simulink model "RudderActuatorChannel_control_linear"  (R2015a)
settings: Solver=ode4  StartTime=0.0  StopTime=2  FixedStep=sampleTime  MaxStep=1e-3  MinStep=1e-4
values from neighbouring files (symbols this model uses):
  StateControl =     [StateControl.mat]
  StateControlLinear =     [StateControlLinear.mat]
undefined symbols (not defined in the file or in its folder): C, ControlTopology, EHSV_Step, Imax, Input, Kd, Ki, Kp, L0, Load_cmd, Max_Cmd, Max_Load_TED, Max_Load_TEU, Min_Cmd, ON_OFF_hyst, OpenLoop, R, Rate_Limit, sampleTime, sigbuilder_block, StiffnessTest_Enable, StiffTest, T_ES, Theta0, Tol_SA1
undefined symbols (not defined in the file): dpLVDT, Kd_N, ramLVDT, xvLVDT
libraries: simulink x3
settings Model: SimulationMode=accelerator  Creator=Charles  LastModifiedBy=Pedro H
settings SolverCC: InitialStep=1e-4
settings DataIOCC: LimitDataPoints=off  SaveFormat=StructureWithTime  DSMLogging=off  SaveTime=off
settings OptimizationCC: ExpressionDepthLimit=2147483647  InitFltsAndDblsToZero=on
settings DebuggingCC: SaveWithParameterizedLinksMsg=none  UnderspecifiedInitializationDetection=Classic  MergeDetectMultiDrivingBlocksExec=none  SolverPrmCheckMsg=warning  InheritedTsInSrcMsg=none  FcnCallInpInsideContextMsg=UseLocalSettings  StateNameClashWarn=warning
settings ModelReferenceCC: UpdateModelReferenceTargets=IfOutOfDate
settings GRTTargetCC: TargetFcnLib=ansi_tfl_tmw.mat  CombineOutputUpdateFcns=off  GRTInterface=on

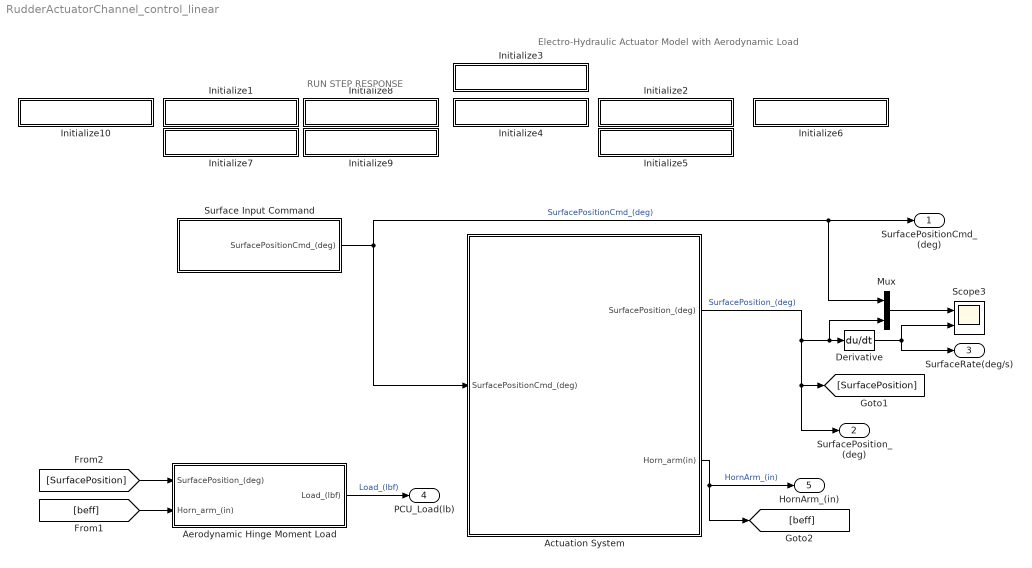
== system RudderActuatorChannel_control_linear ==
  note: RUN STEP RESPONSE
  note: Electro-Hydraulic Actuator Model with Aerodynamic Load
  Actuation System : Subsystem
  Aerodynamic Hinge Moment Load : Subsystem
  Derivative : Derivative  CoefficientInTFapproximation=1e6
  Initialize1 : Subsystem
      settings: OpenFcn=|
      | run('StepInput_CLLoad.m'),
      | set_param(bdroot,'SimulationCommand','start')
      mask Display: disp('Closed Loop - Loaded')
  Initialize10 : Subsystem
      settings: OpenFcn=|
      | run('SineInput_CLLoad.m'),
      | set_param(bdroot,'SimulationCommand','start')
      mask Display: disp('Run Sine Input')
  Initialize2 : Subsystem
      settings: OpenFcn=|
      | FreqResp_type = 0;
      | run('FrequencyResponseTest.m'),
      | set_param(bdroot,'SimulationCommand','start')
      mask Display: disp('Frequency Response')
  Initialize3 : Subsystem
      settings: OpenFcn=run('Load_Parameters.m'),
      mask Display: disp('Model Initialization')
  Initialize4 : Subsystem
      settings: OpenFcn=run('plotMaster.m')
      mask Display: disp('Plot Results')
  Initialize5 : Subsystem
      settings: OpenFcn=|
      | FreqResp_type = 1;
      | run('FrequencyResponseTest.m'),
      | set_param(bdroot,'SimulationCommand','start')
      mask Display: disp('Run EHSV Frequency Response Test')
  Initialize6 : Subsystem
      settings: OpenFcn=run('DynamicStiffnessTest.m')
      mask Display: disp('Dynamic Stiffness Test')
  Initialize7 : Subsystem
      settings: OpenFcn=|
      | run('StepInput_CLNoLoad.m'),
      | set_param(bdroot,'SimulationCommand','start')
      mask Display: disp('Closed Loop - Unloaded')
  Initialize8 : Subsystem
      settings: OpenFcn=|
      | run('StepInput_OLEHSVLoad.m'),
      | set_param(bdroot,'SimulationCommand','start')
      mask Display: disp('Open Loop - Loaded')
  Initialize9 : Subsystem
      settings: OpenFcn=|
      | run('StepInput_OLEHSVNoLoad.m'),
      | set_param(bdroot,'SimulationCommand','start')
      mask Display: disp('Open Loop - Unloaded')
  Mux : Mux  Inputs=2
  Scope3 : Scope  NumInputPorts=2
      settings: TimeRange=3.4  YMin=28.7~-5  YMax=30.8~5  SaveName=Theta
  Surface Input Command : Subsystem
  SurfacePositionCmd_(deg) : Outport
  SurfacePosition_(deg) : Outport  Port=2
  SurfaceRate(deg/s) : Outport  Port=3
  PCU_Load(lb) : Outport  Port=4
  HornArm_(in) : Outport  Port=5
  wires:
  Actuation System/1(SurfacePosition_(deg)) -> SurfacePosition_(deg)/1, [SurfacePosition], Mux/2, Derivative/1  "SurfacePosition_(deg)"
  [SurfacePosition] -> Aerodynamic Hinge Moment Load/1(SurfacePosition_(deg))
  Surface Input Command/1(SurfacePositionCmd_(deg)) -> Mux/1, SurfacePositionCmd_(deg)/1, Actuation System/1(SurfacePositionCmd_(deg))  "SurfacePositionCmd_(deg)"
  Actuation System/2(Horn_arm(in)) -> [beff], HornArm_(in)/1  "HornArm_(in)"
  [beff] -> Aerodynamic Hinge Moment Load/2(Horn_arm_(in))
  Aerodynamic Hinge Moment Load/1(Load_(lbf)) -> PCU_Load(lb)/1  "Load_(lbf)"
  Derivative/1 -> Scope3/2, SurfaceRate(deg/s)/1
  Mux/1 -> Scope3/1

== system RudderActuatorChannel_control_linear/Actuation System ==
  SurfacePositionCmd_(deg) : Inport
  Actuator : Subsystem
  Electronics System : Subsystem
  Surface Kinematics : Subsystem
  SurfacePosition_(deg) : Outport
  Horn_arm(in) : Outport  Port=2
  wires:
  [Sensors_FB] -> Electronics System/2(Sensors_FB)
  SurfacePositionCmd_(deg)/1 -> [Theta_Cmd]
  [Theta_Cmd] -> Electronics System/1(Theta_Cmd_(deg))
  Actuator/1(Xp_real_(in)) -> Surface Kinematics/1(Xp_(in))  "Xp"
  Surface Kinematics/1(ThetaPos_(deg)) -> SurfacePosition_(deg)/1
  Actuator/2(Sensors) -> [Sensors_FB]
  Surface Kinematics/2(Effective_arm_(in)) -> Horn_arm(in)/1
  Electronics System/1(Current_Cmd_(mA)) -> Actuator/1(Current_Cmd)

== system RudderActuatorChannel_control_linear/Aerodynamic Hinge Moment Load ==
  note: Aerodynamic Hinge Moment Load
  SurfacePosition_(deg) : Inport
  Horn_arm_(in) : Inport  Port=2
  1-D Lookup Table : Lookup_n-D  NumberOfTableDimensions=1  BreakpointsForDimension1=[-1 0 1]  Table=[-Max_Load_TED 0 Max_Load_TEU]  RndMeth=Simplest  InputSameDT=on
  Constant : Constant  Value=StiffnessTest_Enable
  Constant1 : Constant  Value=Load_cmd
  Divide : Product  Inputs=*/
  Gain : Gain  Gain=1/Max_Cmd
  Load Type Selector : MultiPortSwitch
  Stiffness Test Load : Sin  Amplitude=StiffTest.Sine_Amplitude  Bias=StiffTest.Sine_Bias  Frequency=StiffTest.Sine_Frequency  SampleTime=0
  Load_(lbf) : Outport
  wires:
  SurfacePosition_(deg)/1 -> Gain/1
  Constant/1 -> Load Type Selector/1
  Gain/1 -> 1-D Lookup Table/1
  Load Type Selector/1 -> Load_(lbf)/1
  Stiffness Test Load/1 -> Load Type Selector/2
  Constant1/1 -> Load Type Selector/4
  1-D Lookup Table/1 -> Divide/1
  Divide/1 -> Load Type Selector/3
  Horn_arm_(in)/1 -> Divide/2

== system RudderActuatorChannel_control_linear/Initialize1 ==

== system RudderActuatorChannel_control_linear/Initialize10 ==

== system RudderActuatorChannel_control_linear/Initialize2 ==

== system RudderActuatorChannel_control_linear/Initialize3 ==

== system RudderActuatorChannel_control_linear/Initialize4 ==

== system RudderActuatorChannel_control_linear/Initialize5 ==

== system RudderActuatorChannel_control_linear/Initialize6 ==

== system RudderActuatorChannel_control_linear/Initialize7 ==

== system RudderActuatorChannel_control_linear/Initialize8 ==

== system RudderActuatorChannel_control_linear/Initialize9 ==

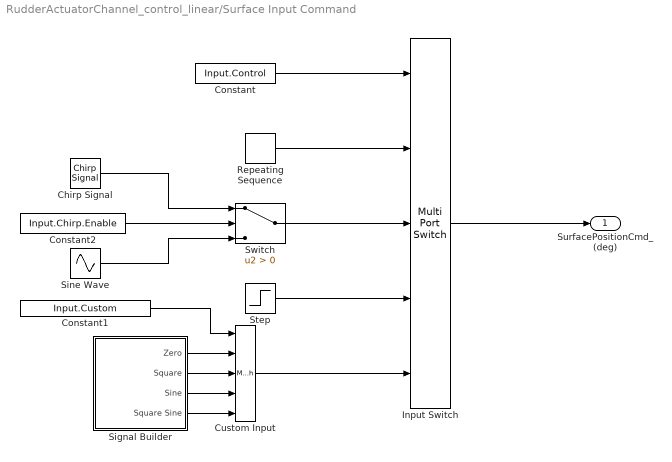
== system RudderActuatorChannel_control_linear/Surface Input Command ==
  Chirp Signal : simulink/Sources/Chirp Signal  f1=Input.Chirp.InitialFrequency  T=Input.Chirp.TargetTime  f2=Input.Chirp.TargetFrequency
  Constant : Constant  Value=Input.Control
  Constant1 : Constant  Value=Input.Custom
  Constant2 : Constant  Value=Input.Chirp.Enable
  Custom Input : MultiPortSwitch  Inputs=4
  Input Switch : MultiPortSwitch  Inputs=4
  Repeating Sequence : simulink/Sources/Repeating Sequence  rep_seq_t=Input.Sequence.Time  rep_seq_y=Input.Sequence.Output
  Signal Builder : Subsystem  Tag=STV Subsys  LoadFcn=sigbuilder_block('load');  StartFcn=sigbuilder_block('start');  StopFcn=sigbuilder_block('stop');  ClipboardFcn=sigbuilder_block('clipboard');  mask(Sigbuilder block){}
      mask help: Simulink:masks:SigbuilderBlock_MD
      mask init:
      | if ~strcmp(get_param(bdroot(gcbh),'SimulationStatus'),'stopped') tuvar = sigbuilder_block('maskInit'); end
      settings: CopyFcn=sigbuilder_block('copy');  DeleteFcn=sigbuilder_block('delete');  ModelCloseFcn=sigbuilder_block('modelClose');  PreSaveFcn=sigbuilder_block('preSave');  PauseFcn=sigbuilder_block('pause');  ContinueFcn=sigbuilder_block('continue');  NameChangeFcn=sigbuilder_block('namechange');  OpenFcn=sigbuilder_block('open',[321.75 116.25 544.5 393.75 ]);  CloseFcn=sigbuilder_block('close');
      mask Display: plot(0, 0, 100, 100,[2, 2, 32, 32, 2], [68, 8, 8, 68, 68],[32, 2], [38, 38], [32, 19, 2],[53, 60, 44], [32, 17, 17, 2],[16, 16, 31, 31]);txt = getActiveGroup(gcbh);text(2, 100, txt,'verticalAlignment', 'top');
  Sine Wave : Sin  Amplitude=Input.Sine.Amplitude  Bias=Input.Sine.Bias  Frequency=Input.Sine.Frequency  Phase=Input.Sine.Phase  SampleTime=0
  Step : Step  Time=Input.Step.Time  Before=Input.Step.InitialValue  After=Input.Step.FinalValue  SampleTime=0
  Switch : Switch  Criteria=u2 > Threshold
  SurfacePositionCmd_(deg) : Outport
  wires:
  Constant/1 -> Input Switch/1
  Input Switch/1 -> SurfacePositionCmd_(deg)/1
  Step/1 -> Input Switch/4
  Switch/1 -> Input Switch/3
  Repeating Sequence/1 -> Input Switch/2
  Custom Input/1 -> Input Switch/5
  Constant1/1 -> Custom Input/1
  Signal Builder/2(Square) -> Custom Input/3
  Signal Builder/1(Zero) -> Custom Input/2
  Signal Builder/3(Sine) -> Custom Input/4
  Signal Builder/4(Square Sine) -> Custom Input/5
  Chirp Signal/1 -> Switch/1
  Sine Wave/1 -> Switch/3
  Constant2/1 -> Switch/2

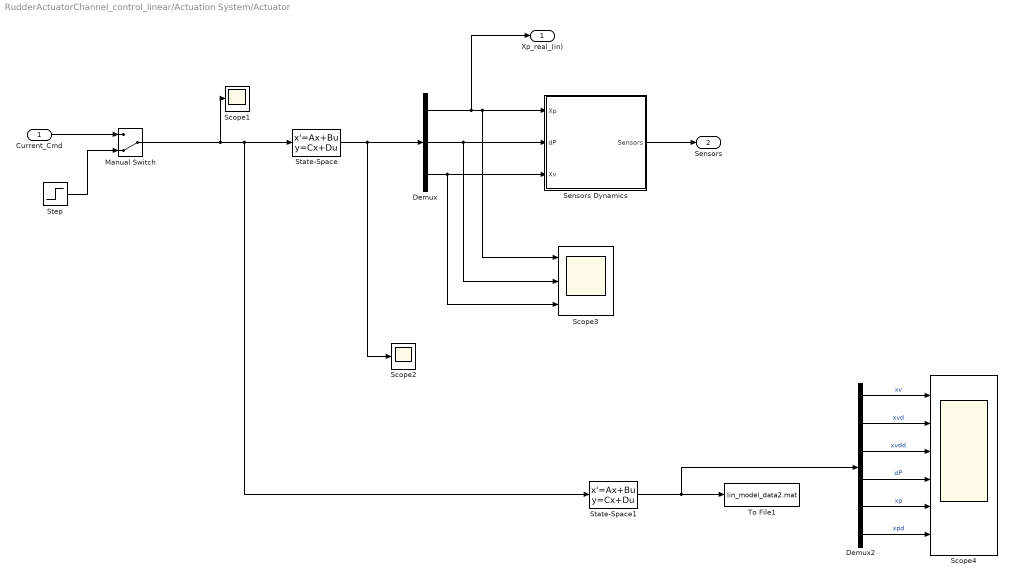
== system RudderActuatorChannel_control_linear/Actuation System/Actuator ==
  Current_Cmd : Inport
  Demux : Demux  Outputs=3
  Demux2 : Demux  Outputs=6
  Manual Switch : ManualSwitch  CurrentSetting=0
  Scope1 : Scope
      settings: SaveName=ScopeData4
  Scope2 : Scope
      settings: SaveName=ScopeData5
  Scope3 : Scope  NumInputPorts=3
      settings: YMin=-5~-5~-5  YMax=5~5~5  SaveName=ScopeData3
  Scope4 : Scope  NumInputPorts=6
      settings: TimeRange=1.515675675675676  YMin=-5.9091e-26~-400000~0~-6.08696e-06~-1.15432e-20~-5e-06  YMax=0.0671053~200000~300000~3.3913e-05~0.04~5e-06  SaveName=ScopeData8
  Sensors Dynamics : Subsystem
  State-Space : StateSpace  A=StateControl.A  B=StateControl.B  C=StateControlLinear.C  D=zeros(3,1)  X0=StateControl.X0
  State-Space1 : StateSpace  A=StateControl.A  B=StateControl.B  C=eye(6)  D=zeros(6,1)  X0=StateControl.X0
  Step : Step  Time=0.5  After=4  SampleTime=0
  To File1 : ToFile  Filename=lin_model_data2.mat  MatrixName=states_lin  SaveFormat=Timeseries
  Xp_real_(in) : Outport
  Sensors : Outport  Port=2
  wires:
  Sensors Dynamics/1(Sensors) -> Sensors/1
  State-Space/1 -> Scope2/1, Demux/1
  Demux/3 -> Scope3/3, Sensors Dynamics/3(Xv)
  Demux/1 -> Xp_real_(in)/1, Scope3/1, Sensors Dynamics/1(Xp)
  Demux/2 -> Scope3/2, Sensors Dynamics/2(dP)
  Current_Cmd/1 -> Manual Switch/1
  Manual Switch/1 -> Scope1/1, State-Space1/1, State-Space/1
  Step/1 -> Manual Switch/2
  State-Space1/1 -> Demux2/1, To File1/1
  Demux2/5 -> Scope4/5  "xp"
  Demux2/4 -> Scope4/4  "dP"
  Demux2/3 -> Scope4/3  "xvdd"
  Demux2/1 -> Scope4/1  "xv"
  Demux2/2 -> Scope4/2  "xvd"
  Demux2/6 -> Scope4/6  "xpd"

== system RudderActuatorChannel_control_linear/Actuation System/Electronics System ==
  Theta_Cmd_(deg) : Inport
  Sensors_FB : Inport  Port=2
  Analog Controller : Subsystem
  Constant : Constant  Value=ControlTopology
  Digital Controller : Subsystem
  Hardware_in : Subsystem
  Hardware_out : Subsystem
  Switch : Switch  Threshold=5.5
  Current_Cmd_(mA) : Outport
  wires:
  Theta_Cmd_(deg)/1 -> Analog Controller/1(Cmd_D), Hardware_in/1(Theta_Cmd_in)
  Digital Controller/1(EHSV_Cmd) -> Hardware_out/1(EHSV_Cmd_in)
  Hardware_out/1(EHSV_Cmd_out) -> Switch/3  "Current_Cmd_CL"
  Hardware_in/1(Theta_Cmd_out) -> Digital Controller/1(Cmd_D)
  Hardware_in/2(Sensors_FB_out) -> Digital Controller/2(Sensors_FB)
  Sensors_FB/1 -> Analog Controller/2(Sensors_FB), Hardware_in/2(Sensors_FB_in)
  Switch/1 -> Current_Cmd_(mA)/1
  Analog Controller/1(EHSV_Cmd) -> Switch/1
  Constant/1 -> Switch/2

== system RudderActuatorChannel_control_linear/Actuation System/Surface Kinematics ==
  Xp_(in) : Inport
  Rad2Deg : Gain  Gain=180/pi  SaturateOnIntegerOverflow=on  OutDataTypeStr=Inherit: Same as input  ParamDataTypeStr=Inherit: Same as input
  Real Kinematics : Subsystem
  ThetaPos_(deg) : Outport
  Effective_arm_(in) : Outport  Port=2
  wires:
  Xp_(in)/1 -> Real Kinematics/1(Xp)
  Real Kinematics/1(Theta) -> Rad2Deg/1
  Rad2Deg/1 -> ThetaPos_(deg)/1
  Real Kinematics/2(Reff) -> Effective_arm_(in)/1

== system RudderActuatorChannel_control_linear/Surface Input Command/Signal Builder ==
  Demux : Demux  Tag=STV Demux
  FromWs : FromWorkspace  Tag=STV FromWs  VariableName=tuvar  SampleTime=0
      SigBuilderData=|
      | common.afterFinalStr = 'Extrapolate'
      | common.sampleTime = 0
      | dataSet.timeRange = [0 10]
      | dataSet.name = 'Group 1'
      | sbobj.Groups.Name = 'Group 1'
      | sbobj.Groups.Signals(1).Name = 'Zero'
      | sbobj.Groups.Signals(1).XData = [0 10]
      | sbobj.Groups.Signals(1).YData = [0 0]
      | sbobj.Groups.Signals(2).Name = 'Square'
      | sbobj.Groups.Signals(2).XData = [0 4 4 6 6 10]
      | sbobj.Groups.Signals(2).YData = [0 0 1 1 0 0]
      | sbobj.Groups.Signals(3).Name = 'Sine'
      | sbobj.Groups.Signals(3).XData = [0 0.125 0.25 0.375 0.5 0.625 0.75 0.875 1 1.125 1.25 1.375 1.5 1.625 1.75 1.875 2 2.125 2.25 2.375 2.5 2.625 2.75 2.875 3 3.125 3.25 3.375 3.5 3.625 3.75 3.875 4 4.125 4.25 4.375 4.5 4.625 4.75 4.875 5 5.125 5.25 5.375 5.5 5.625 5.75 5.875 6 6.125 6.25 6.375 6.5 6.625 6.75 6.875 7 7.125 7.25 7.375 7.5 7.625 7.75 7.875 8 8.125 8.25 8.375 8.5 8.625 8.75 8.875 9 9.125 9.25 9.375 9.5 9.625 9.75 9.875 10]
      | sbobj.Groups.Signals(3).YData = [1 1.70710678119 2 1.70710678119 1 0.292893218813 0 0.292893218813 1 1.70710678119 2 1.70710678119 1 0.292893218813 0 0.292893218813 1 1.70710678119 2 1.70710678119 1 0.292893218813 0 0.292893218813 1 1.70710678119 2 1.70710678119 1 0.292893218813 0 0.292893218813 1 1.70710678119 2 1.70710678119 1 0.292893218813 0 0.292893218813 1 1.70710678119 2 1.70710678119 1 0.292893218813 0 0.292893218813 1 1.70710678119 2 1.70710678119 1 0.292893218813 0 0.292893218813 1 1.70710678119 2 1.70710678119 1 0.292893218813 0 0.292893218813 1 1.70710678119 2 1.70710678119 1 0.292893218813 0 0.292893218813 1 1.70710678119 2 1.70710678119 1 0.292893218813 0 0.292893218813 1]
      | sbobj.Groups.Signals(4).Name = 'Square Sine'
      | sbobj.Groups.Signals(4).XData = [0 0.5 0.5 1 1 1.5 1.5 2 2 2.5 2.5 3 3 3.5 3.5 4 4 4.5 4.5 5 5 5.5 5.5 6 6 6.5 6.5 7 7 7.5 7.5 8 8 8.5 8.5 9 9 9.5 9.5 10]
      | sbobj.Groups.Signals(4).YData = [2 2 0 0 2 2 0 0 2 2 0 0 2 2 0 0 2 2 0 0 2 2 0 0 2 2 0 0 2 2 0 0 2 2 0 0 2 2 0 0]
  Zero : Outport  Tag=STV Outport
  Square : Outport  Tag=STV Outport  Port=2
  Sine : Outport  Tag=STV Outport  Port=3
  Square Sine : Outport  Tag=STV Outport  Port=4
  wires:
  FromWs/1 -> Demux/1
  Demux/1 -> Zero/1
  Demux/2 -> Square/1
  Demux/3 -> Sine/1
  Demux/4 -> Square Sine/1

== system RudderActuatorChannel_control_linear/Actuation System/Actuator/Sensors Dynamics ==
  Xp : Inport
  dP : Inport  Port=2
  Xv : Inport  Port=3
  Bus Creator : BusCreator  Inputs=3
  "Xp LVDT " : Subsystem
  "Xv LVDT " : Subsystem
  "dP LVDT " : Subsystem
  Sensors : Outport
  wires:
  dP/1 -> "dP LVDT "/1(dP_real)
  Xp/1 -> "Xp LVDT "/1(Xp_real)
  Xv/1 -> "Xv LVDT "/1(Xv_real)
  "Xv LVDT "/1(Xv_LVDT) -> Bus Creator/3  "Xv_mesured_(in)"
  "dP LVDT "/1(dP_LVDT) -> Bus Creator/2  "dP_mesured_(psi)"
  "Xp LVDT "/1(Xp_LVDT) -> Bus Creator/1  "Xp_mesured_(in)"
  Bus Creator/1 -> Sensors/1

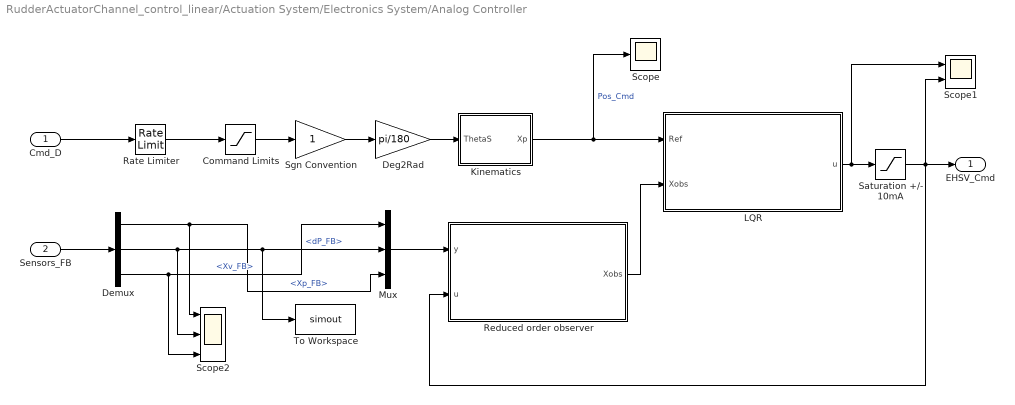
== system RudderActuatorChannel_control_linear/Actuation System/Electronics System/Analog Controller ==
  Cmd_D : Inport
  Sensors_FB : Inport  Port=2
  Command Limits : Saturate  UpperLimit=Max_Cmd  LowerLimit=Min_Cmd
  Deg2Rad : Gain  Gain=pi/180  SaturateOnIntegerOverflow=on  OutDataTypeStr=Inherit: Same as input  ParamDataTypeStr=Inherit: Same as input
  Demux : Demux  Outputs=3
  Kinematics : Subsystem
  LQR : Subsystem  mask{K=[14.6507   -0.0011   -0.0000    0.0003   22.9112   -0.0053]}
      mask prompts: K "State Control gain (K)"
  Mux : Mux  Inputs=3
  Rate Limiter : RateLimiter  RisingSlewLimit=Rate_Limit*0.9  FallingSlewLimit=-Rate_Limit*0.9  SampleTimeMode=inherited
  Reduced order observer : Subsystem  mask{H=StateControl.Obs.H, A=StateControl.Obs.A, K=StateControl.Obs.K, L=StateControl.Obs.L}
      mask prompts: H "H obs"; A "A obs"; K "K obs"; L "L obs"
  Saturation +/- 10mA : Saturate  UpperLimit=Imax  LowerLimit=-Imax
  Scope : Scope
      settings: TimeRange=3  YMin=0  YMax=3.5  SaveName=ScopeData9
  Scope1 : Scope  NumInputPorts=2
      settings: YMin=-5~-5  YMax=5~5  SaveName=ScopeData10
  Scope2 : Scope  NumInputPorts=3
      settings: YMin=-5~-5~-5  YMax=5~5~5  SaveName=ScopeData11
  Sgn Convention : Gain  SaturateOnIntegerOverflow=on  OutDataTypeStr=Inherit: Same as input  ParamDataTypeStr=Inherit: Same as input
  To Workspace : ToWorkspace  VariableName=simout  SaveFormat=Timeseries  SampleTime=-1
  EHSV_Cmd : Outport
  wires:
  Cmd_D/1 -> Rate Limiter/1
  Kinematics/1(Xp) -> Scope/1, LQR/1(Ref)  "Pos_Cmd"
  Command Limits/1 -> Sgn Convention/1
  Deg2Rad/1 -> Kinematics/1(ThetaS)
  Rate Limiter/1 -> Command Limits/1
  Sgn Convention/1 -> Deg2Rad/1
  Sensors_FB/1 -> Demux/1
  Demux/1 -> Scope2/1, Mux/3  "<Xp_FB>"
  Demux/2 -> Scope2/2, Mux/2, To Workspace/1  "<dP_FB>"
  Demux/3 -> Scope2/3, Mux/1  "<Xv_FB>"
  Mux/1 -> Reduced order observer/1(y)
  Reduced order observer/1(Xobs) -> LQR/2(Xobs)
  LQR/1(u) -> Scope1/1, Saturation +/- 10mA/1
  Saturation +/- 10mA/1 -> Reduced order observer/2(u), Scope1/2, EHSV_Cmd/1

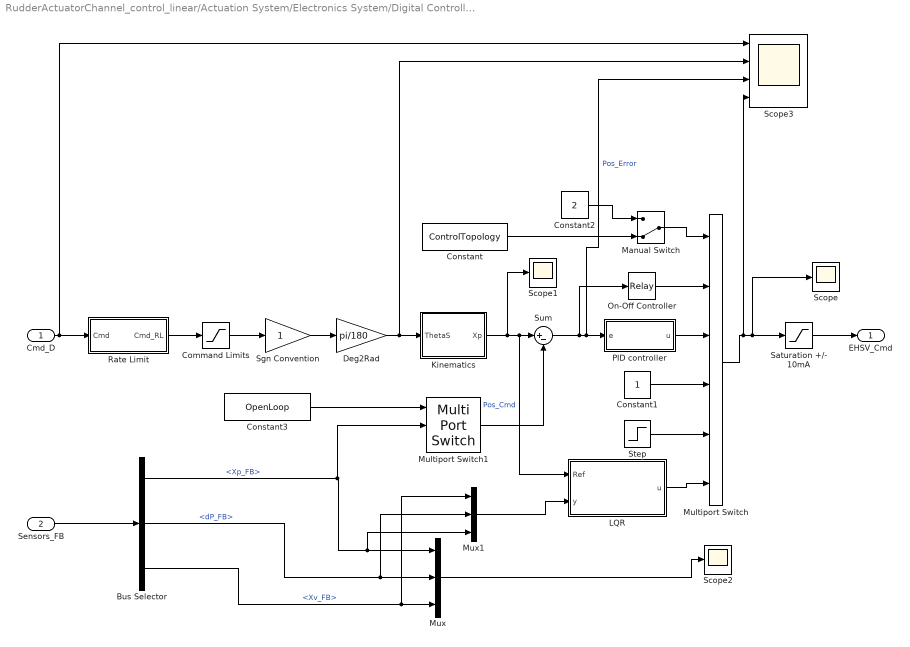
== system RudderActuatorChannel_control_linear/Actuation System/Electronics System/Digital Controller ==
  Cmd_D : Inport
  Sensors_FB : Inport  Port=2
  Bus Selector : BusSelector  OutputSignals=Xp_FB,dP_FB,Xv_FB
  Command Limits : Saturate  UpperLimit=Max_Cmd  LowerLimit=Min_Cmd
  Constant : Constant  Value=ControlTopology
  Constant1 : Constant
  Constant2 : Constant  Value=2
  Constant3 : Constant  Value=OpenLoop
  Deg2Rad : Gain  Gain=pi/180  SampleTime=T_ES  SaturateOnIntegerOverflow=on  OutDataTypeStr=Inherit: Same as input  ParamDataTypeStr=Inherit: Same as input
  Kinematics : Subsystem
  LQR : Subsystem  mask{K=[14.6507 0.0003   22.9112 ]}
      mask prompts: K "State Control gain (K)"
  Manual Switch : ManualSwitch  CurrentSetting=0
  Multiport Switch : MultiPortSwitch  Inputs=5
  Multiport Switch1 : MultiPortSwitch  DataPortOrder=Zero-based contiguous  Inputs=2
  Mux : Mux  Inputs=3
  Mux1 : Mux  Inputs=3
  On-Off Controller : Relay  OnSwitchValue=ON_OFF_hyst  OffSwitchValue=-ON_OFF_hyst  OnOutputValue=10  OffOutputValue=-10
  PID controller : Subsystem  mask{Kp=Kp, Ki=Ki, Kd=Kd, Ts=T_ES, kd_N=Kd_N, umax=10}
      mask prompts: Ts "Sampling Time"; kd_N "Kd Filter coefficient"; umax "Max command"
  Rate Limit : Subsystem
  Saturation +/- 10mA : Saturate  UpperLimit=Imax  LowerLimit=-Imax  SampleTime=T_ES
  Scope : Scope
  Scope1 : Scope
      settings: SaveName=ScopeData2
  Scope2 : Scope
      settings: SaveName=ScopeData7
  Scope3 : Scope  NumInputPorts=4
      settings: YMin=-5~-5~-5~-5  YMax=5~5~5~5
  Sgn Convention : Gain  SampleTime=T_ES  SaturateOnIntegerOverflow=on  OutDataTypeStr=Inherit: Same as input  ParamDataTypeStr=Inherit: Same as input
  Step : Step  Time=EHSV_Step.time  Before=EHSV_Step.initial  After=EHSV_Step.final
  Sum : Sum  Inputs=|+-  SampleTime=T_ES  SaturateOnIntegerOverflow=on  InputSameDT=on  OutDataTypeStr=Inherit: Same as first input
  EHSV_Cmd : Outport
  wires:
  Cmd_D/1 -> Scope3/1, Rate Limit/1(Cmd)
  Kinematics/1(Xp) -> Scope1/1, LQR/1(Ref), Sum/1  "Pos_Cmd"
  Saturation +/- 10mA/1 -> EHSV_Cmd/1
  Sum/1 -> On-Off Controller/1, Scope3/3, PID controller/1(e)  "Pos_Error"
  Command Limits/1 -> Sgn Convention/1
  Deg2Rad/1 -> Scope3/2, Kinematics/1(ThetaS)
  Rate Limit/1(Cmd_RL) -> Command Limits/1
  Sgn Convention/1 -> Deg2Rad/1
  Sensors_FB/1 -> Bus Selector/1
  Bus Selector/1 -> Multiport Switch1/2, Mux1/3, Mux/1  "<Xp_FB>"
  Bus Selector/2 -> Mux1/2, Mux/2  "<dP_FB>"
  Bus Selector/3 -> Mux1/1, Mux/3  "<Xv_FB>"
  Multiport Switch/1 -> Scope3/4, Scope/1, Saturation +/- 10mA/1
  Constant/1 -> Manual Switch/2
  On-Off Controller/1 -> Multiport Switch/2
  Constant1/1 -> Multiport Switch/4
  PID controller/1(u) -> Multiport Switch/3
  Step/1 -> Multiport Switch/5
  Mux/1 -> Scope2/1
  Manual Switch/1 -> Multiport Switch/1
  Constant2/1 -> Manual Switch/1
  Mux1/1 -> LQR/2(y)
  LQR/1(u) -> Multiport Switch/6
  Multiport Switch1/1 -> Sum/2
  Constant3/1 -> Multiport Switch1/1

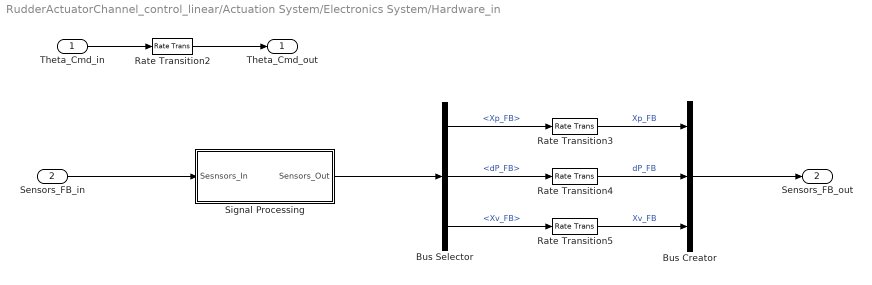
== system RudderActuatorChannel_control_linear/Actuation System/Electronics System/Hardware_in ==
  Theta_Cmd_in : Inport
  Sensors_FB_in : Inport  Port=2
  Bus Creator : BusCreator  Inputs=3
  Bus Selector : BusSelector  OutputSignals=Xp_FB,dP_FB,Xv_FB
  Rate Transition{2..5} (4 alike) : RateTransition  Deterministic=off  OutPortSampleTime=T_ES
  Signal Processing : Subsystem
  Theta_Cmd_out : Outport
  Sensors_FB_out : Outport  Port=2
  wires:
  Bus Creator/1 -> Sensors_FB_out/1
  Theta_Cmd_in/1 -> Rate Transition2/1
  Rate Transition2/1 -> Theta_Cmd_out/1
  Sensors_FB_in/1 -> Signal Processing/1(Sesnsors_In)
  Bus Selector/1 -> Rate Transition3/1  "<Xp_FB>"
  Rate Transition3/1 -> Bus Creator/1  "Xp_FB"
  Rate Transition4/1 -> Bus Creator/2  "dP_FB"
  Rate Transition5/1 -> Bus Creator/3  "Xv_FB"
  Bus Selector/2 -> Rate Transition4/1  "<dP_FB>"
  Bus Selector/3 -> Rate Transition5/1  "<Xv_FB>"
  Signal Processing/1(Sensors_Out) -> Bus Selector/1

== system RudderActuatorChannel_control_linear/Actuation System/Electronics System/Hardware_out ==
  EHSV_Cmd_in : Inport
  Rate Transition : RateTransition  Deterministic=off  OutPortSampleTime=0
  Servoamplifier Dynamics : TransferFcn  Numerator=[100]  Denominator=[1 100]
  Servoamplifier Tolerance : Gain  Gain=Tol_SA1
  EHSV_Cmd_out : Outport
  wires:
  Rate Transition/1 -> Servoamplifier Dynamics/1
  Servoamplifier Dynamics/1 -> Servoamplifier Tolerance/1
  EHSV_Cmd_in/1 -> Rate Transition/1
  Servoamplifier Tolerance/1 -> EHSV_Cmd_out/1  "Current"

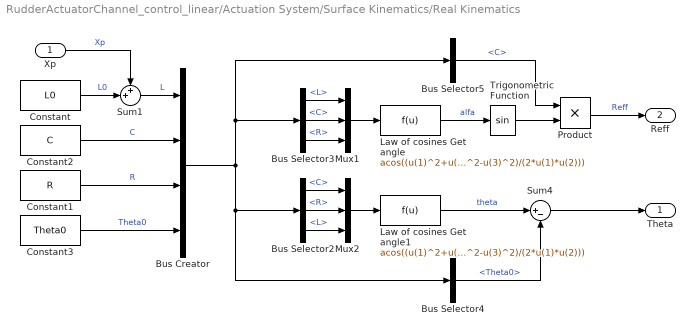
== system RudderActuatorChannel_control_linear/Actuation System/Surface Kinematics/Real Kinematics ==
  Xp : Inport
  Bus Creator : BusCreator
  Bus Selector2 : BusSelector  OutputSignals=C,R,L
  Bus Selector3 : BusSelector  OutputSignals=L,C,R
  Bus Selector4 : BusSelector  OutputSignals=Theta0
  Bus Selector5 : BusSelector  OutputSignals=C
  Constant : Constant  Value=L0
  Constant1 : Constant  Value=R
  Constant2 : Constant  Value=C
  Constant3 : Constant  Value=Theta0
  Law of cosines Get angle : Fcn  Expr=acos((u(1)^2+u(2)^2-u(3)^2)/(2*u(1)*u(2)))
  Law of cosines Get angle1 : Fcn  Expr=acos((u(1)^2+u(2)^2-u(3)^2)/(2*u(1)*u(2)))
  Mux1 : Mux  Inputs=3
  Mux2 : Mux  Inputs=3
  Product : Product  RndMeth=Zero
  Sum1 : Sum  Inputs=++|
  Sum4 : Sum  Inputs=|+-
  Trigonometric Function : Trigonometry
  Theta : Outport
  Reff : Outport  Port=2
  wires:
  Mux2/1 -> Law of cosines Get angle1/1
  Bus Selector2/1 -> Mux2/1  "<C>"
  Bus Selector2/2 -> Mux2/2  "<R>"
  Law of cosines Get angle1/1 -> Sum4/1  "theta"
  Bus Selector4/1 -> Sum4/2  "<Theta0>"
  Sum4/1 -> Theta/1
  Xp/1 -> Sum1/1  "Xp"
  Constant/1 -> Sum1/2  "L0"
  Sum1/1 -> Bus Creator/1  "L"
  Constant2/1 -> Bus Creator/2  "C"
  Constant1/1 -> Bus Creator/3  "R"
  Constant3/1 -> Bus Creator/4  "Theta0"
  Mux1/1 -> Law of cosines Get angle/1
  Law of cosines Get angle/1 -> Trigonometric Function/1  "alfa"
  Bus Selector3/1 -> Mux1/1  "<L>"
  Bus Selector3/2 -> Mux1/2  "<C>"
  Bus Selector3/3 -> Mux1/3  "<R>"
  Product/1 -> Reff/1  "Reff"
  Bus Selector5/1 -> Product/1  "<C>"
  Trigonometric Function/1 -> Product/2
  Bus Selector2/3 -> Mux2/3  "<L>"
  Bus Creator/1 -> Bus Selector3/1, Bus Selector5/1, Bus Selector2/1, Bus Selector4/1

== system RudderActuatorChannel_control_linear/Actuation System/Actuator/Sensors Dynamics/Xp LVDT  ==
  Xp_real : Inport
  LVDT : Subsystem  mask{band=ramLVDT.Bandwidth, range=ramLVDT.Range, lvdt_error=ramLVDT.Error, hyst=ramLVDT.Hysteresis}
      mask prompts: band "LVDT Bandwdidth"; range "LVDT Range ([min middle max])"; lvdt_error "LVDT error"; hyst "LVDT Hysteresis"
  Xp_LVDT : Outport
  wires:
  Xp_real/1 -> LVDT/1(Sensor In)
  LVDT/1(SensorOut) -> Xp_LVDT/1

== system RudderActuatorChannel_control_linear/Actuation System/Actuator/Sensors Dynamics/Xv LVDT  ==
  Xv_real : Inport
  LVDT1 : Subsystem  mask{band=xvLVDT.Bandwidth, range=xvLVDT.Range, lvdt_error=xvLVDT.Error, hyst=xvLVDT.Hysteresis}
      mask prompts: band "LVDT Bandwdidth (Hz)"; range "LVDT Range ([min middle max])"; lvdt_error "LVDT error"; hyst "LVDT Hysteresis (%)"
  Xv_LVDT : Outport
  wires:
  Xv_real/1 -> LVDT1/1(Sensor In)
  LVDT1/1(SensorOut) -> Xv_LVDT/1

== system RudderActuatorChannel_control_linear/Actuation System/Actuator/Sensors Dynamics/dP LVDT  ==
  dP_real : Inport
  LVDT1 : Subsystem  mask{band=dpLVDT.Bandwidth, range=dpLVDT.Range, lvdt_error=dpLVDT.Error, hyst=dpLVDT.Hysteresis}
      mask prompts: band "LVDT Bandwdidth (Hz)"; range "LVDT Range ([min middle max])"; lvdt_error "LVDT error"; hyst "LVDT Hysteresis (%)"
  dP_LVDT : Outport
  wires:
  dP_real/1 -> LVDT1/1(Sensor In)
  LVDT1/1(SensorOut) -> dP_LVDT/1

== system RudderActuatorChannel_control_linear/Actuation System/Electronics System/Analog Controller/Kinematics ==
  ThetaS : Inport
  Constant : Constant  Value=L0
  Constant1 : Constant  Value=R
  Constant2 : Constant  Value=C
  Constant3 : Constant  Value=Theta0
  Law of cosines Get side : Fcn  Expr=sqrt(u(1)^2+u(2)^2-2*u(1)*u(2)*cos(u(3)))
  Mux1 : Mux  Inputs=3
  Sum : Sum  Inputs=|++
  Sum1 : Sum  Inputs=|+-
  Xp : Outport
  wires:
  Constant2/1 -> Mux1/1  "C"
  Constant1/1 -> Mux1/2  "R"
  Mux1/1 -> Law of cosines Get side/1
  ThetaS/1 -> Sum/1  "ThetaS"
  Sum/1 -> Mux1/3
  Law of cosines Get side/1 -> Sum1/1  "L"
  Constant/1 -> Sum1/2  "L0"
  Sum1/1 -> Xp/1
  Constant3/1 -> Sum/2  "Theta0"

== system RudderActuatorChannel_control_linear/Actuation System/Electronics System/Analog Controller/LQR ==
  Ref : Inport
  Xobs : Inport  Port=2
  Add : Sum  Inputs=|+-
  Add1 : Sum  Inputs=|+-
  Demux1 : Demux  Outputs=6
  Gain : Gain  Gain=K(5)
  Gain1 : Gain  Gain=[K(1:4) K(6)]./K(5)  Multiplication=Matrix(K*u) (u vector)
  Mux : Mux  Inputs=5
  u : Outport
  wires:
  Xobs/1 -> Demux1/1
  Demux1/6 -> Mux/5
  Demux1/4 -> Mux/4
  Demux1/3 -> Mux/3
  Demux1/2 -> Mux/2
  Demux1/1 -> Mux/1
  Ref/1 -> Add/1
  Demux1/5 -> Add/2
  Add/1 -> Add1/1
  Mux/1 -> Gain1/1
  Add1/1 -> Gain/1
  Gain/1 -> u/1
  Gain1/1 -> Add1/2

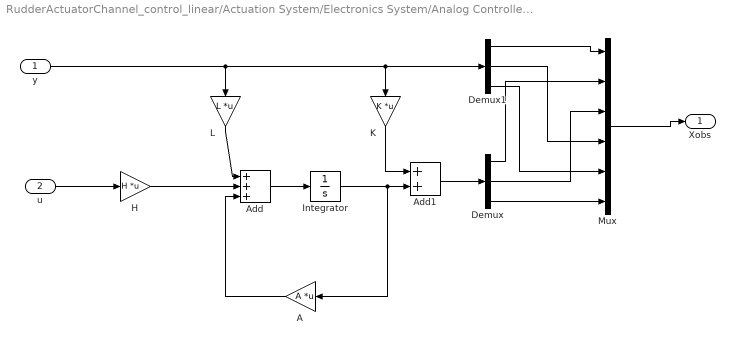
== system RudderActuatorChannel_control_linear/Actuation System/Electronics System/Analog Controller/Reduced order observer ==
  y : Inport
  u : Inport  Port=2
  A : Gain  Gain=A  Multiplication=Matrix(K*u)
  Add : Sum  Inputs=+++
  Add1 : Sum
  Demux : Demux  Outputs=3
  Demux1 : Demux  Outputs=3
  H : Gain  Gain=H  Multiplication=Matrix(K*u)
  Integrator : Integrator
  K : Gain  Gain=K  Multiplication=Matrix(K*u)
  L : Gain  Gain=L  Multiplication=Matrix(K*u)
  Mux : Mux  Inputs=6
  Xobs : Outport
  wires:
  y/1 -> Demux1/1, K/1, L/1
  H/1 -> Add/2
  u/1 -> H/1
  A/1 -> Add/3
  L/1 -> Add/1
  Add/1 -> Integrator/1
  Integrator/1 -> A/1, Add1/2
  K/1 -> Add1/1
  Add1/1 -> Demux/1
  Demux1/1 -> Mux/1
  Demux1/2 -> Mux/4
  Demux1/3 -> Mux/5
  Demux/1 -> Mux/2
  Demux/2 -> Mux/3
  Demux/3 -> Mux/6
  Mux/1 -> Xobs/1

== system RudderActuatorChannel_control_linear/Actuation System/Electronics System/Digital Controller/Kinematics ==
  ThetaS : Inport
  Constant : Constant  Value=L0
  Constant1 : Constant  Value=R
  Constant2 : Constant  Value=C
  Constant3 : Constant  Value=Theta0
  Law of cosines Get side : Fcn  Expr=sqrt(u(1)^2+u(2)^2-2*u(1)*u(2)*cos(u(3)))  SampleTime=T_ES
  Mux1 : Mux  Inputs=3
  Sum : Sum  Inputs=|++  SampleTime=T_ES
  Sum1 : Sum  Inputs=|+-  SampleTime=T_ES
  Xp : Outport
  wires:
  Constant2/1 -> Mux1/1  "C"
  Constant1/1 -> Mux1/2  "R"
  Mux1/1 -> Law of cosines Get side/1
  ThetaS/1 -> Sum/1  "ThetaS"
  Sum/1 -> Mux1/3
  Law of cosines Get side/1 -> Sum1/1  "L"
  Constant/1 -> Sum1/2  "L0"
  Sum1/1 -> Xp/1
  Constant3/1 -> Sum/2  "Theta0"

== system RudderActuatorChannel_control_linear/Actuation System/Electronics System/Digital Controller/LQR ==
  Ref : Inport
  y : Inport  Port=2
  Add : Sum  Inputs=|+-
  Add1 : Sum  Inputs=|+-
  Demux1 : Demux  Outputs=3
  Gain : Gain  Gain=K(3)
  Gain1 : Gain  Gain=[K(1) K(2)]./K(3)  Multiplication=Matrix(K*u) (u vector)
  Input control : Scope  NumInputPorts=2
      settings: TimeRange=1.515675675675676  YMin=-5.9091e-26~-400000  YMax=0.0671053~200000  SaveName=ScopeData6
  Mux : Mux  Inputs=2
  u : Outport
  wires:
  y/1 -> Demux1/1
  Ref/1 -> Add/1
  Add/1 -> Input control/1, Add1/1
  Mux/1 -> Gain1/1
  Add1/1 -> Input control/2, Gain/1
  Gain/1 -> u/1
  Gain1/1 -> Add1/2
  Demux1/1 -> Mux/1
  Demux1/2 -> Mux/2
  Demux1/3 -> Add/2

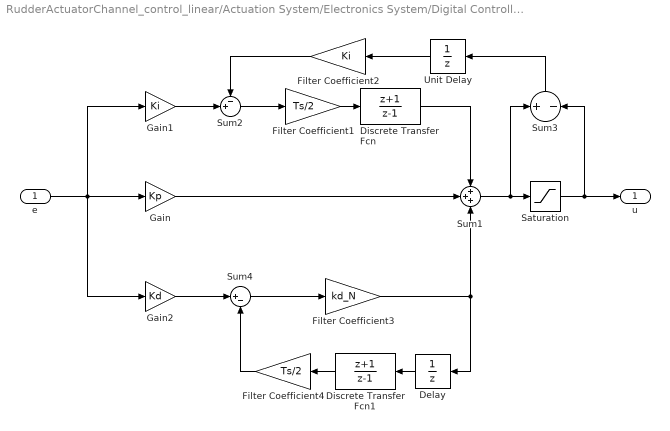
== system RudderActuatorChannel_control_linear/Actuation System/Electronics System/Digital Controller/PID controller ==
  e : Inport
  Delay : UnitDelay  SampleTime=-1
  Discrete Transfer Fcn : DiscreteTransferFcn  Numerator=[1 1]  Denominator=[1 -1]
  Discrete Transfer Fcn1 : DiscreteTransferFcn  Numerator=[1 1]  Denominator=[1 -1]
  Filter Coefficient1 : Gain  Gain=Ts/2
  Filter Coefficient2 : Gain  Gain=Ki
  Filter Coefficient3 : Gain  Gain=kd_N
  Filter Coefficient4 : Gain  Gain=Ts/2
  Gain : Gain  Gain=Kp
  Gain1 : Gain  Gain=Ki
  Gain2 : Gain  Gain=Kd
  "Saturation " : Saturate  UpperLimit=umax  LowerLimit=-umax  SampleTime=T_ES
  Sum1 : Sum  Inputs=+++
  Sum2 : Sum  Inputs=-+|
  Sum3 : Sum  Inputs=+-
  Sum4 : Sum  Inputs=|+-
  Unit Delay : UnitDelay  SampleTime=-1
  u : Outport
  wires:
  Gain1/1 -> Sum2/2
  Gain/1 -> Sum1/2
  Sum1/1 -> Sum3/1, "Saturation "/1
  e/1 -> Gain2/1, Gain/1, Gain1/1
  Discrete Transfer Fcn/1 -> Sum1/1
  Filter Coefficient1/1 -> Discrete Transfer Fcn/1
  Gain2/1 -> Sum4/1
  Sum2/1 -> Filter Coefficient1/1
  "Saturation "/1 -> u/1, Sum3/2
  Sum3/1 -> Unit Delay/1
  Filter Coefficient2/1 -> Sum2/1
  Unit Delay/1 -> Filter Coefficient2/1
  Sum4/1 -> Filter Coefficient3/1
  Discrete Transfer Fcn1/1 -> Filter Coefficient4/1
  Filter Coefficient4/1 -> Sum4/2
  Delay/1 -> Discrete Transfer Fcn1/1
  Filter Coefficient3/1 -> Sum1/3, Delay/1

== system RudderActuatorChannel_control_linear/Actuation System/Electronics System/Digital Controller/Rate Limit ==
  Cmd : Inport
  Gain : Gain  Gain=1/T_ES
  Gain1 : Gain  Gain=T_ES
  Rate Limit : Saturate  UpperLimit=Rate_Limit  LowerLimit=-Rate_Limit
  Sum3 : Sum  Inputs=|+-  SaturateOnIntegerOverflow=on  InputSameDT=on  OutDataTypeStr=Inherit: Same as first input
  Sum4 : Sum  Inputs=|++  SaturateOnIntegerOverflow=on  InputSameDT=on  OutDataTypeStr=Inherit: Same as first input
  Unit Delay1 : UnitDelay  SampleTime=-1
  Unit Delay2 : UnitDelay  SampleTime=-1
  Cmd_RL : Outport
  wires:
  Cmd/1 -> Sum3/1
  Unit Delay1/1 -> Sum3/2
  Sum3/1 -> Gain/1  "dCmd"
  Gain/1 -> Rate Limit/1  "Rate"
  Rate Limit/1 -> Gain1/1  "Rate Limited"
  Unit Delay2/1 -> Sum4/2
  Sum4/1 -> Unit Delay2/1, Cmd_RL/1, Unit Delay1/1
  Gain1/1 -> Sum4/1

== system RudderActuatorChannel_control_linear/Actuation System/Electronics System/Hardware_in/Signal Processing ==
  Sesnsors_In : Inport
  Add1 : Sum
  Band-Limited White Noise : simulink/Sources/Band-Limited White Noise  Cov=[0.5]  Ts=sampleTime  seed=[23341]
  Bus Creator : BusCreator  Inputs=3
  Bus Selector : BusSelector  OutputSignals=Xp_mesured_(in),dP_mesured_(psi),Xv_mesured_(in)
  RAM LVDT Tolerance : Gain
  Xv LVDT Tolerance : Gain
  dp LVDT Tolerance : Gain
  Sensors_Out : Outport
  wires:
  Sesnsors_In/1 -> Bus Selector/1
  Bus Selector/3 -> Xv LVDT Tolerance/1  "<Xv_mesured_(in)>"
  Bus Selector/1 -> RAM LVDT Tolerance/1  "<Xp_mesured_(in)>"
  Bus Selector/2 -> Add1/1  "<dP_mesured_(psi)>"
  RAM LVDT Tolerance/1 -> Bus Creator/1  "Xp_FB"
  dp LVDT Tolerance/1 -> Bus Creator/2  "dP_FB"
  Xv LVDT Tolerance/1 -> Bus Creator/3  "Xv_FB"
  Bus Creator/1 -> Sensors_Out/1
  Band-Limited White Noise/1 -> Add1/2
  Add1/1 -> dp LVDT Tolerance/1

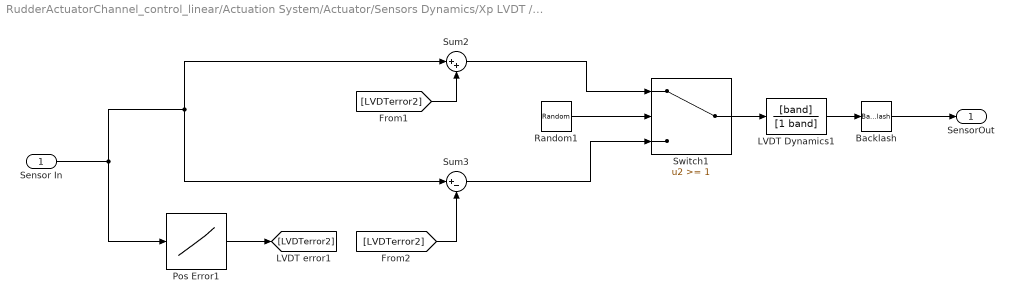
== system RudderActuatorChannel_control_linear/Actuation System/Actuator/Sensors Dynamics/Xp LVDT /LVDT ==
  Sensor In : Inport
  " Pos Error1" : Lookup_n-D  NumberOfTableDimensions=1  BreakpointsForDimension1=[range(1) range(2) range(3)]  Table=[lvdt_error lvdt_error*0.4 lvdt_error]  RndMeth=Simplest  InputSameDT=on
  Backlash : Backlash  BacklashWidth=(range(3)-range(2))*hyst/100
  LVDT Dynamics1 : TransferFcn  Numerator=[band]  Denominator=[1 band]
  Random1 : RandomNumber  Mean=1  Variance=10
  Sum2 : Sum  Inputs=|++
  Sum3 : Sum  Inputs=|+-
  Switch1 : Switch  Threshold=1
  SensorOut : Outport
  wires:
  [LVDTerror2] -> Sum3/2
  Switch1/1 -> LVDT Dynamics1/1
  Sum2/1 -> Switch1/1
  Sensor In/1 -> Sum2/1, Sum3/1, " Pos Error1"/1
  Random1/1 -> Switch1/2
  [LVDTerror2] -> Sum2/2
  Sum3/1 -> Switch1/3
  " Pos Error1"/1 -> [LVDTerror2]
  LVDT Dynamics1/1 -> Backlash/1
  Backlash/1 -> SensorOut/1

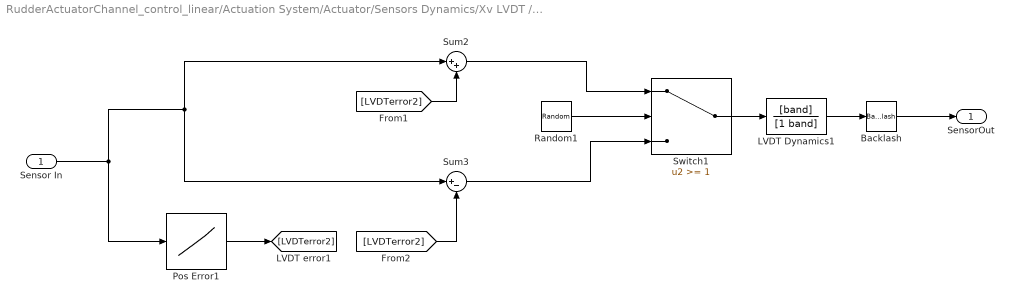
== system RudderActuatorChannel_control_linear/Actuation System/Actuator/Sensors Dynamics/Xv LVDT /LVDT1 ==
  Sensor In : Inport
  " Pos Error1" : Lookup_n-D  NumberOfTableDimensions=1  BreakpointsForDimension1=[range(1) range(2) range(3)]  Table=[lvdt_error lvdt_error*0.4 lvdt_error]  RndMeth=Simplest  InputSameDT=on
  Backlash : Backlash  BacklashWidth=(range(3)-range(2))*hyst/100
  LVDT Dynamics1 : TransferFcn  Numerator=[band]  Denominator=[1 band]
  Random1 : RandomNumber  Mean=1  Variance=10
  Sum2 : Sum  Inputs=|++
  Sum3 : Sum  Inputs=|+-
  Switch1 : Switch  Threshold=1
  SensorOut : Outport
  wires:
  [LVDTerror2] -> Sum3/2
  Switch1/1 -> LVDT Dynamics1/1
  Sum2/1 -> Switch1/1
  Sensor In/1 -> Sum2/1, Sum3/1, " Pos Error1"/1
  Random1/1 -> Switch1/2
  [LVDTerror2] -> Sum2/2
  Sum3/1 -> Switch1/3
  " Pos Error1"/1 -> [LVDTerror2]
  LVDT Dynamics1/1 -> Backlash/1
  Backlash/1 -> SensorOut/1

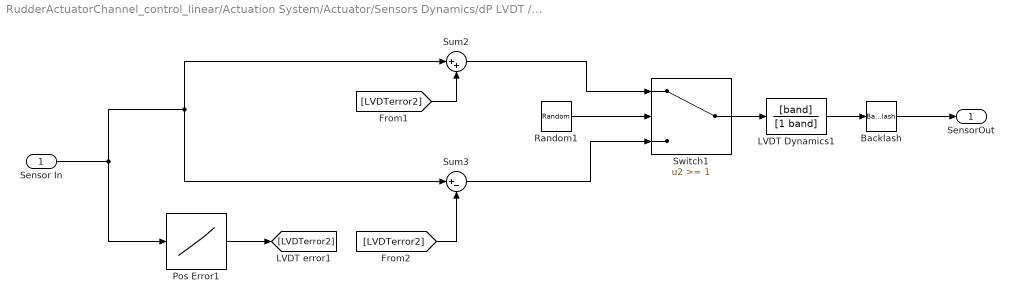
== system RudderActuatorChannel_control_linear/Actuation System/Actuator/Sensors Dynamics/dP LVDT /LVDT1 ==
  Sensor In : Inport
  " Pos Error1" : Lookup_n-D  NumberOfTableDimensions=1  BreakpointsForDimension1=[range(1) range(2) range(3)]  Table=[lvdt_error lvdt_error*0.4 lvdt_error]  RndMeth=Simplest  InputSameDT=on
  Backlash : Backlash  BacklashWidth=(range(3)-range(2))*hyst/100
  LVDT Dynamics1 : TransferFcn  Numerator=[band]  Denominator=[1 band]
  Random1 : RandomNumber  Mean=1  Variance=10
  Sum2 : Sum  Inputs=|++
  Sum3 : Sum  Inputs=|+-
  Switch1 : Switch  Threshold=1
  SensorOut : Outport
  wires:
  [LVDTerror2] -> Sum3/2
  Switch1/1 -> LVDT Dynamics1/1
  Sum2/1 -> Switch1/1
  Sensor In/1 -> Sum2/1, Sum3/1, " Pos Error1"/1
  Random1/1 -> Switch1/2
  [LVDTerror2] -> Sum2/2
  Sum3/1 -> Switch1/3
  " Pos Error1"/1 -> [LVDTerror2]
  LVDT Dynamics1/1 -> Backlash/1
  Backlash/1 -> SensorOut/1
